simulink model "rlattempt1"  (R2022b)
settings: Solver=FixedStepDiscrete  StartTime=0.0  StopTime=inf  RelTol=1e-3
values from neighbouring files (symbols this model uses):
  mapSize = 10    [main.m]
libraries: rllib x1
settings Model: Creator=88692  LastModifiedBy=w7474
settings DebuggingCC: AlgebraicLoopMsg=none  UnconnectedInputMsg=warning  UnconnectedOutputMsg=warning  UnconnectedLineMsg=warning
settings ModelReferenceCC: EnableRefExpFcnMdlSchedulingChecks=on
settings SFSimCC: SimTargetLang=C++  GPUAcceleration=on  SimGPUStackLimitPerThread=2048  SimDLTargetLibrary=cudnn
settings RTWCC: DLArmComputeVersion=19.05

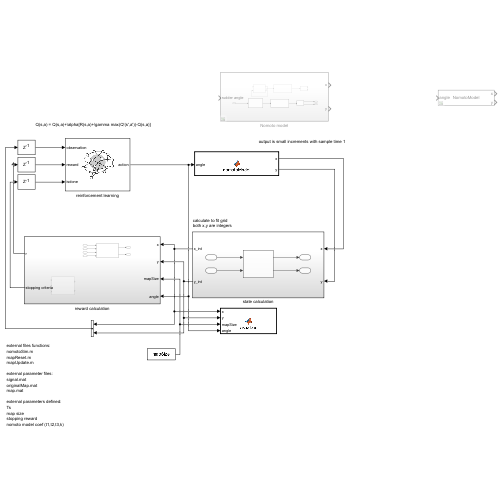
[thumbnail: Simulink's stored preview of the top-level diagram]
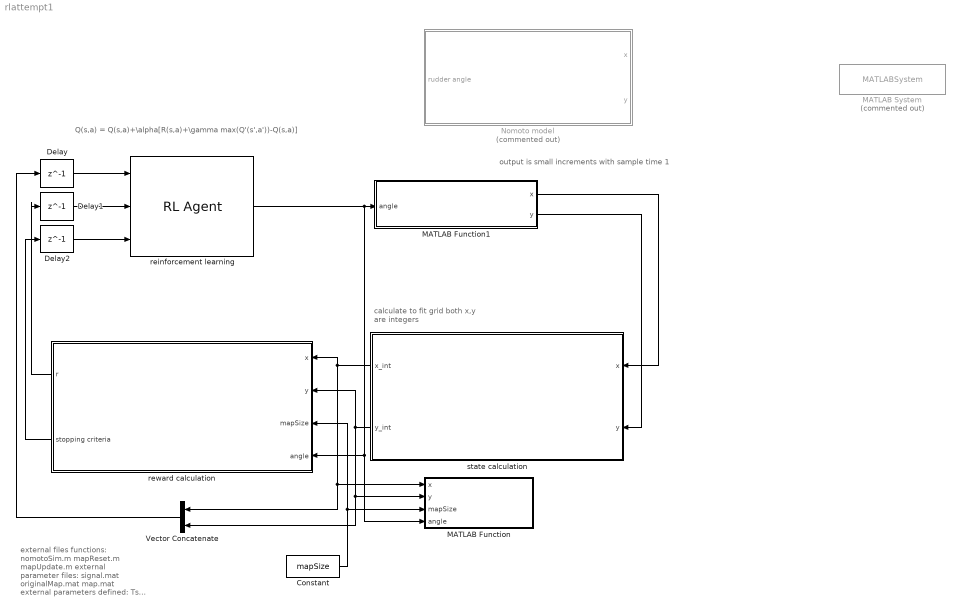
== system rlattempt1 ==
  note: external files functions:
      | nomotoSim.m
      | mapReset.m
      | mapUpdate.m
      |
      | external parameter files:
      | signal.mat
      | originalMap.mat
      | map.mat
      |
      | external parameters defined:
      | Ts
      | map size
      | stopping reward
      | nomoto model coef (t1,t2,t3,k)
  note: Q(s,a) = Q(s,a)+\alpha[R(s,a)+\gamma max(Q'(s',a'))-Q(s,a)]
  note: calculate to fit grid
      | both x,y are integers
  note: output is small increments with sample time 1
  Constant : Constant  Value=mapSize
  Delay : Delay  DelayLength=1  InitialCondition=0
  Delay1 : Delay  DelayLength=1  InitialCondition=0
  Delay2 : Delay  DelayLength=1  InitialCondition=0
  MATLAB Function : MATLAB Function  TreatAsAtomicUnit=on
  MATLAB Function1 : MATLAB Function  TreatAsAtomicUnit=on
  MATLAB System : MATLABSystem  Commented=on  System=NomotoModel  Ts=1  SimulateUsing=Code generation
      mask Type: NomotoModel
      mask Display:
      | disp('NomotoModel');
      | port_label('input',1,'angle');
      | port_label('output',1,'x');
      | port_label('output',2,'y');
  Nomoto model : Subsystem  Commented=on
  Vector Concatenate : Concatenate
  reinforcement learning : rllib/RL Agent  Agent=agent  ExternalActionAsInput=off  ProvideLastAction=off  ProvideCumRwd=off  TreatAsDirectFeedthrough=on  UseStrictObservationDataTypes=off
  reward calculation : Subsystem
  state calculation : Subsystem
  wires:
  state calculation/1(x_int) -> Vector Concatenate/1, MATLAB Function/1(x), reward calculation/1(x)
  state calculation/2(y_int) -> Vector Concatenate/2, MATLAB Function/2(y), reward calculation/2(y)
  MATLAB Function1/1(x) -> state calculation/1(x)
  reward calculation/1(r) -> Delay1/1
  Vector Concatenate/1 -> Delay/1
  reward calculation/2(stopping criteria) -> Delay2/1
  MATLAB Function1/2(y) -> state calculation/2(y)
  Delay2/1 -> reinforcement learning/3
  Delay1/1 -> reinforcement learning/2
  Delay/1 -> reinforcement learning/1
  Constant/1 -> reward calculation/3(mapSize), MATLAB Function/3(mapSize)
  reinforcement learning/1 -> MATLAB Function1/1(angle), reward calculation/4(angle), MATLAB Function/4(angle)

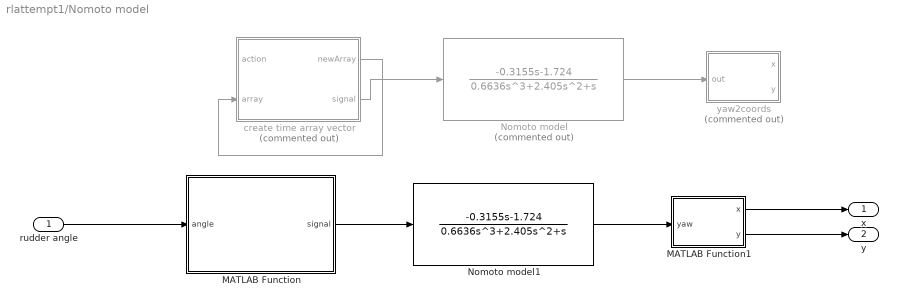
== system rlattempt1/Nomoto model ==
  rudder angle : Inport
  MATLAB Function : MATLAB Function  TreatAsAtomicUnit=on
  MATLAB Function1 : MATLAB Function  TreatAsAtomicUnit=on
  Nomoto model : TransferFcn  Commented=on  Numerator=[-0.3155 -1.724]  Denominator=[0.6636 2.405 1 0]
  Nomoto model1 : TransferFcn  Numerator=[-0.3155 -1.724]  Denominator=[0.6636 2.405 1 0]
  create time array vector : MATLAB Function  Commented=on  TreatAsAtomicUnit=on
  yaw2coords : MATLAB Function  Commented=on  TreatAsAtomicUnit=on
  x : Outport
  y : Outport  Port=2
  wires:
  Nomoto model/1 -> yaw2coords/1(out)
  rudder angle/1 -> MATLAB Function/1(angle)
  create time array vector/1(newArray) -> create time array vector/2(array)
  create time array vector/2(signal) -> Nomoto model/1
  MATLAB Function/1(signal) -> Nomoto model1/1
  Nomoto model1/1 -> MATLAB Function1/1(yaw)
  MATLAB Function1/1(x) -> x/1
  MATLAB Function1/2(y) -> y/1

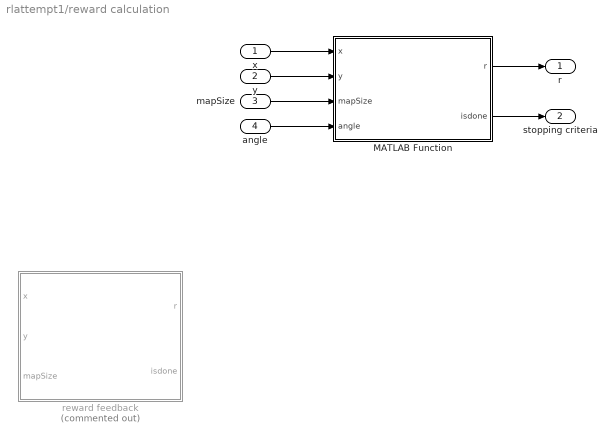
== system rlattempt1/reward calculation ==
  x : Inport
  y : Inport  Port=2
  mapSize : Inport  Port=3
  angle : Inport  Port=4
  MATLAB Function : MATLAB Function  TreatAsAtomicUnit=on
  reward feedback : MATLAB Function  Commented=on  TreatAsAtomicUnit=on
  r : Outport
  stopping criteria : Outport  Port=2
  wires:
  x/1 -> MATLAB Function/1(x)
  y/1 -> MATLAB Function/2(y)
  mapSize/1 -> MATLAB Function/3(mapSize)
  MATLAB Function/2(isdone) -> stopping criteria/1
  MATLAB Function/1(r) -> r/1
  angle/1 -> MATLAB Function/4(angle)

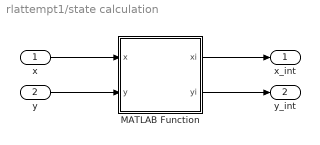
== system rlattempt1/state calculation ==
  x : Inport
  y : Inport  Port=2
  MATLAB Function : MATLAB Function  TreatAsAtomicUnit=on
  x_int : Outport
  y_int : Outport  Port=2
  wires:
  x/1 -> MATLAB Function/1(x)
  y/1 -> MATLAB Function/2(y)
  MATLAB Function/1(xi) -> x_int/1
  MATLAB Function/2(yi) -> y_int/1

== matlab function rlattempt1/Nomoto model/create time array vector ==
  data: action input; newArray output; array input; signal output
function [newArray, signal]= time(action, array)
    newArray = [array action];
    signal = array2timetable(newArray, 'SampleRate', 100);
end

== matlab function rlattempt1/Nomoto model/yaw2coords ==
  data: x output; out input; y output
function [x,y] = fcn(out)
    longchange = cos(out)*0.02;
    latchange = sin(out)*0.02;
    y = zeros(1,length(longchange));
    x = zeros(1,length(latchange));
    for i = 2:length(out)
        y(i) = y(i-1) + longchange(i-1);
        x(i) = x(i-1) + latchange(i-1);
    end
[x,y] = u;

== matlab function rlattempt1/reward calculation/reward feedback ==
  data: x input; r output; y input; isdone output; mapSize input
function [r,isdone] = reward(x,y,mapSize)
    % reward is equivalent to number of oysters - weight*time passed
    coder.extrinsic('mapUpdate');
    oysters = 0;
    mapMatrix = 50*ones(mapSize,mapSize);
    [oysters, mapMatrix] = mapUpdate(x,y,mapSize);
    r = oysters-1;
    isdone = sum(mapMatrix,'all') <= 500;
end

== matlab function rlattempt1/MATLAB Function1 ==
  data: x output; y output; angle input
function [x,y] = nomotoModel(angle)
    x = 0;
    y = 0;
    coder.extrinsic('nomotoSim');
    [x,y] = nomotoSim(angle);
end

== matlab function rlattempt1/state calculation/MATLAB Function ==
  data: x input; xi output; y input; yi output
function [xi,yi]= floor(x,y)
    % Nomoto Model coordinates start at (0,0) and is a floating point
    % state is constricted to a map starting at (1,1) integer
    xi = floor(x)+1;
    yi = floor(y)+1;
end

== matlab function rlattempt1/Nomoto model/MATLAB Function ==
  data: angle input; signal output
function signal = fcn(angle)
    s = load("signal.mat");
    currentSignal = s.newArray;
    newArray = [currentSignal angle];
    signal = array2timetable(newArray, 'SampleRate', 100);
    save("signal.mat","newArray");    
end

== matlab function rlattempt1/Nomoto model/MATLAB Function1 ==
  data: x output; yaw input; y output
function [x,y]= fcn(yaw)
    longchange = cos(yaw)*0.02;
    latchange = sin(yaw)*0.02;
    yout = zeros(1,length(longchange));
    xout = zeros(1,length(latchange));
    for i = 2:length(yaw)
        yout(i) = yout(i-1) + longchange(i-1);
        xout(i) = xout(i-1) + latchange(i-1);
    end

    x = xout(length(xout));
    y = yout(length(yout));
end

== matlab function rlattempt1/MATLAB Function ==
  data: x input; y input; mapSize input; angle input
function visualizer(x,y,mapSize,angle)
    coder.extrinsic("visualizer");
    visualizer(x,y,mapSize,angle);

== matlab function rlattempt1/reward calculation/MATLAB Function ==
  data: x input; r output; y input; isdone output; mapSize input; angle input
function [r,isdone] = reward(x,y,mapSize,angle)
    % reward is equivalent to number of oysters - weight*time passed
    coder.extrinsic('rewardCal');
    oysters = 0;
    isdone = 0;
    [oysters, done] = rewardCal(x,y,mapSize,angle);
    r = oysters;
    isdone = double(done);
end
